simulink model "Method_1_Jerk_Based"  (R2020b)
settings: Solver=VariableStepAuto  StartTime=0.0  StopTime=320  RelTol=1e-3
values from neighbouring files (symbols this model uses):
  GR = 5    [Model_Data.mat]
  m = 220    [Model_Data.mat]
  r = 0.3059    [Model_Data.mat]
  s2_5_rps = [0 104.6666667 209.3333333 314 418.6666667 523.3333333 628]    [Model_Data.mat]
  s2_5_trq = [70 65 60 50 40 33 27]    [Model_Data.mat]
undefined symbols (not defined in the file or in its folder): h, km, s, sigbuilder_block
libraries: autolibshared x4, aerolibconvert2 x2, autolibmappedmotor x1, simulink x1
(part 3 of 3)

== matlab function Method_1_Jerk_Based/Traction Controller ==
  data: Jerk input; acc_out output; Driver_Command input
function acc_out  = fcn(Jerk,Driver_Command)

if (Jerk<1000)
    acc_out = Driver_Command;
end

if (Jerk>1000 && Jerk<5000)
    acc_out = 0.8*Driver_Command;
end

if (Jerk>5000 && Jerk<10000000000)
    acc_out = 0.6*Driver_Command;
end

if (Jerk>10000000000)
    acc_out = 0.4*Driver_Command;

else
    acc_out = Driver_Command;
end

            
 end
